simulink model "Question3_part_f"  (R2020b)
settings: Solver=VariableStepAuto  StartTime=0.0  StopTime=20  RelTol=1e-3
model workspace (MAT data in the model file):
  n1 = 300
  n2 = 200
  y1_init = 400
  y2_init = 100
settings Model: Creator=merih  LastModifiedBy=merih

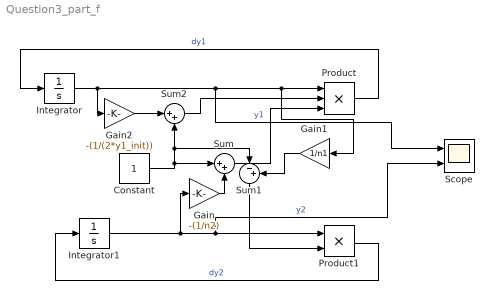
== system Question3_part_f ==
  Constant : Constant
  Gain : Gain  Gain=-(1/n2)
  Gain1 : Gain  Gain=1/n1
  Gain2 : Gain  Gain=-(1/(2*y1_init))
  Integrator : Integrator  InitialCondition=y1_init
  Integrator1 : Integrator  InitialCondition=y2_init
  Product : Product  Inputs=3
  Product1 : Product
  Scope : Scope  NumInputPorts=2
  Sum : Sum  Inputs=|++
  Sum1 : Sum  Inputs=|-+
  Sum2 : Sum  Inputs=|++
  wires:
  Integrator/1 -> Gain2/1, Scope/1, Gain1/1, Product/1  "y1"
  Integrator1/1 -> Gain/1, Scope/2, Product1/1  "y2"
  Gain/1 -> Sum/2
  Constant/1 -> Sum2/2, Sum1/1, Sum/1
  Sum/1 -> Product/3
  Gain1/1 -> Sum1/2
  Sum1/1 -> Product1/2
  Product1/1 -> Integrator1/1  "dy2"
  Product/1 -> Integrator/1  "dy1"
  Gain2/1 -> Sum2/1
  Sum2/1 -> Product/2
